simulink model "ManipRoboticoTraiettoriaspazioOperativo"  (R2025b)
settings: Solver=VariableStepAuto  StartTime=0.0  StopTime=10  RelTol=1e-3
values from neighbouring files (symbols this model uses):
  Kd = [15; 15]    [main.m]
  Kp = [20; 20]    [main.m]
settings Model: Creator=arman  LastModifiedBy=arman

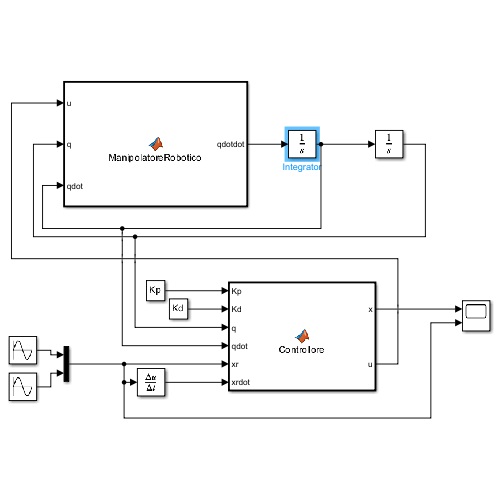
[thumbnail: Simulink's stored preview of the top-level diagram]
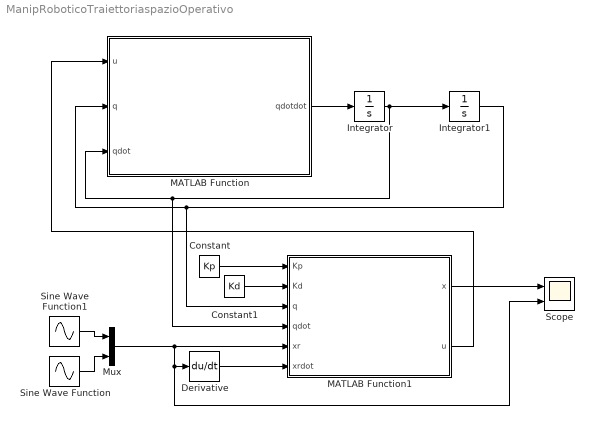
== system ManipRoboticoTraiettoriaspazioOperativo ==
  Constant : Constant  Value=Kp
  Constant1 : Constant  Value=Kd
  Derivative : Derivative
  Integrator : Integrator  InitialCondition=[0;0]
  Integrator1 : Integrator  InitialCondition=[0;0]
  MATLAB Function : MATLAB Function  TreatAsAtomicUnit=on
  MATLAB Function1 : MATLAB Function  TreatAsAtomicUnit=on
  Mux : Mux  Inputs=2
  Scope : Scope  NumInputPorts=2
      settings: ActiveDisplayYMinimum=-2.9765585079799348  ActiveDisplayYMaximum=6.6640620564422157
  Sine Wave Function : Sin  Amplitude=2  SampleTime=0
  Sine Wave Function1 : Sin  Amplitude=2  Phase=pi/2  SampleTime=0
  wires:
  Integrator/1 -> MATLAB Function/3(qdot), MATLAB Function1/4(qdot), Integrator1/1
  MATLAB Function/1(qdotdot) -> Integrator/1
  Integrator1/1 -> MATLAB Function1/3(q), MATLAB Function/2(q)
  MATLAB Function1/2(u) -> MATLAB Function/1(u)
  Constant/1 -> MATLAB Function1/1(Kp)
  Constant1/1 -> MATLAB Function1/2(Kd)
  MATLAB Function1/1(x) -> Scope/1
  Sine Wave Function1/1 -> Mux/1
  Sine Wave Function/1 -> Mux/2
  Mux/1 -> Derivative/1, Scope/2, MATLAB Function1/5(xr)
  Derivative/1 -> MATLAB Function1/6(xrdot)

== matlab function ManipRoboticoTraiettoriaspazioOperativo/MATLAB Function1 ==
  data: x output; Kp input; u output; Kd input; q input; qdot input; xr input; xrdot input
function [x,u] = Controllore(Kp,Kd,q,qdot,xr,xrdot)

[B, C, g, F] = calculateMatrixRobotRR(q,qdot);

l1=3;
l2=2.7;
J = [-l1*sin(q(1))-l2*sin(q(1)+q(2))    -l2*sin(q(1)+q(2));
    l1*cos(q(1)) + l2*cos(q(1)+q(2))    l2*cos(q(1)+ q(2))];

x = [l1*cos(q(1)) + l2*cos(q(1)+q(2));
     l1*sin(q(1)) + l2*sin(q(1)+q(2))];
xdot = J * qdot;
e = x - xr;
edot = xdot - xrdot;
u = g - J.'*(Kd.*edot + Kp.*e);

== matlab function ManipRoboticoTraiettoriaspazioOperativo/MATLAB Function ==
  data: u input; qdotdot output; q input; qdot input
function qdotdot = ManipolatoreRobotico(u,q,qdot)
[B, C, g, F] = calculateMatrixRobotRR(q,qdot);
qdotdot = B \ (u - (C * qdot) - g - F);
